simulink model "Test"  (R2018b)
settings: Solver=ode8  StartTime=0.0  StopTime=100.0  FixedStep=0.01  RelTol=1e-6
undefined symbols (not defined in the file or in its folder): tollerableriskTest_Exists
settings Model: SimulationMode=accelerator  Creator=claudio.menghi  LastModifiedBy=claudio.menghi
settings SolverCC: MaxConsecutiveZCs=10000  ShapePreserveControl=EnableAll  ZeroCrossControl=EnableAll  ZeroCrossAlgorithm=Adaptive  AutoInsertRateTranBlk=on

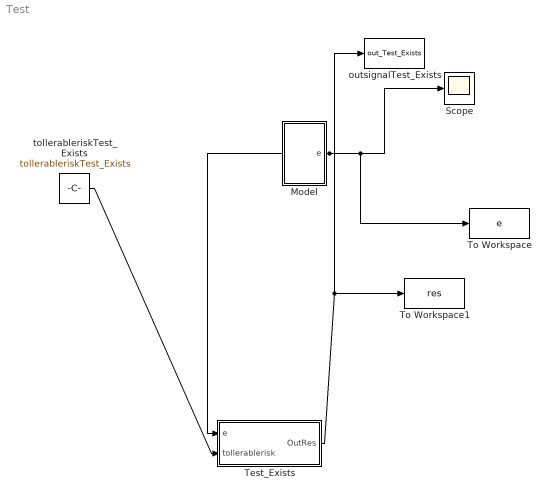
== system Test ==
  Model : Subsystem
  Scope : Scope
  Test_Exists : Subsystem
  To Workspace : ToWorkspace  VariableName=e  SaveFormat=Timeseries  SampleTime=-1
  To Workspace1 : ToWorkspace  VariableName=res  SaveFormat=Timeseries  SampleTime=-1
  outsignalTest_Exists : ToWorkspace  VariableName=out_Test_Exists  SaveFormat=Timeseries  SampleTime=-1
      settings: MaxDataPoints=1
  tollerableriskTest_Exists : Constant  Value=tollerableriskTest_Exists
  wires:
  Model/1(e) -> To Workspace/1, Scope/1, Test_Exists/1(e)
  tollerableriskTest_Exists/1 -> Test_Exists/2(tollerablerisk)
  Test_Exists/1(OutRes) -> To Workspace1/1, outsignalTest_Exists/1

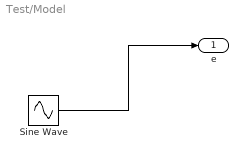
== system Test/Model ==
  Sine Wave : Sin  Amplitude=0.5  SampleTime=0
  e : Outport
  wires:
  Sine Wave/1 -> e/1

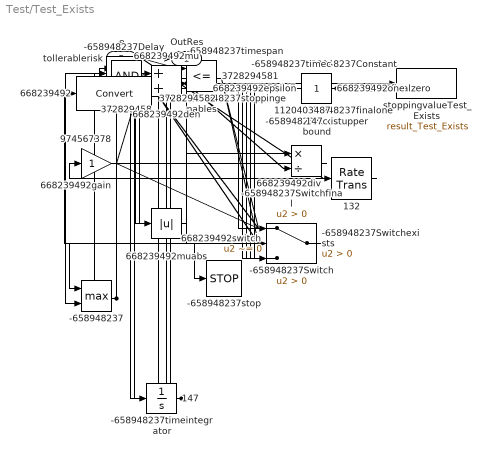
== system Test/Test_Exists ==
  e : Inport
  tollerablerisk : Inport  Port=2
  -658948237 : MinMax  Function=max  Inputs=2
  -658948237Constant : Constant  Value=-1
  -658948237Delay : UnitDelay  InitialCondition=-1  SampleTime=-1
  -658948237Switch : Switch  Criteria=u2 > Threshold
  -658948237Switchexists : Switch  Criteria=u2 > Threshold
  -658948237Switchfinal : Switch  Criteria=u2 > Threshold
  -658948237existupperbound : Constant  Value=100.0
  -658948237finalone : Constant
  -658948237finalzero : Constant  Value=0
  -658948237stop : Stop
  -658948237stoppingenables : RelationalOperator  OutDataTypeStr=boolean  RndMeth=Simplest
  -658948237timec : Constant
  -658948237timeintegrator : Integrator
  -658948237timespan : RelationalOperator  OutDataTypeStr=boolean  RndMeth=Simplest
  1065353247 : Constant  Value=1.0
  1120403487 : Constant  Value=100.0
  132 : RateTransition
  147 : Integrator
  147c : Constant
  31 : Constant  Value=0.0
  372829458 : Logic  AllPortsSameDT=off  OutDataTypeStr=boolean
  3728294581 : RelationalOperator  Operator=<=  OutDataTypeStr=boolean  RndMeth=Simplest
  3728294582 : RelationalOperator  Operator=<=  OutDataTypeStr=boolean  RndMeth=Simplest
  668239492 : DataTypeConversion
  668239492den : Sum
  668239492div : Product  Inputs=*/
  668239492epsilon : Constant  Value=-0.01
  668239492gain : Gain
  668239492mu : Sum  Inputs=+-
  668239492muabs : Abs
  668239492one : Constant
  668239492switch : Switch  Criteria=u2 ~= 0
  974567378 : Gain
  stoppingvalueTest_Exists : ToWorkspace  VariableName=result_Test_Exists  SaveFormat=Timeseries  SampleTime=-1
      settings: MaxDataPoints=1
  OutRes : Outport
  wires:
  147c/1 -> 147/1
  31/1 -> 3728294581/1
  147/1 -> 3728294581/2, 3728294582/1
  1120403487/1 -> 3728294582/2
  3728294581/1 -> 372829458/1
  3728294582/1 -> 372829458/2
  e/1 -> 132/1
  132/1 -> 974567378/1
  974567378/1 -> 668239492mu/1
  1065353247/1 -> 668239492mu/2
  668239492mu/1 -> 668239492muabs/1, 668239492div/1, 668239492switch/2
  668239492muabs/1 -> 668239492den/1
  668239492one/1 -> 668239492den/2
  668239492den/1 -> 668239492div/2
  668239492div/1 -> 668239492gain/1
  668239492gain/1 -> 668239492switch/1
  668239492epsilon/1 -> 668239492switch/3
  668239492switch/1 -> 668239492/1
  -658948237Constant/1 -> -658948237Switch/3
  372829458/1 -> -658948237Switch/2
  668239492/1 -> -658948237Switch/1
  -658948237Switch/1 -> -658948237/1
  -658948237/1 -> -658948237Delay/1, OutRes/1, -658948237timespan/2, stoppingvalueTest_Exists/1
  -658948237Delay/1 -> -658948237/2
  tollerablerisk/1 -> -658948237timespan/1
  -658948237finalzero/1 -> -658948237Switchfinal/3, -658948237Switchexists/3
  -658948237timec/1 -> -658948237timeintegrator/1
  -658948237timeintegrator/1 -> -658948237stoppingenables/1
  -658948237existupperbound/1 -> -658948237stoppingenables/2
  -658948237stoppingenables/1 -> -658948237Switchexists/2
  -658948237timespan/1 -> -658948237Switchexists/1
  -658948237finalone/1 -> -658948237Switchfinal/1
  -658948237Switchexists/1 -> -658948237Switchfinal/2
  -658948237Switchfinal/1 -> -658948237stop/1
